simulink model "Car"  (R2016b)
settings: Solver=VariableStepAuto  StartTime=0.0  StopTime=10.0  RelTol=1e-3
settings Model: Creator=Takiya  LastModifiedBy=Takiya

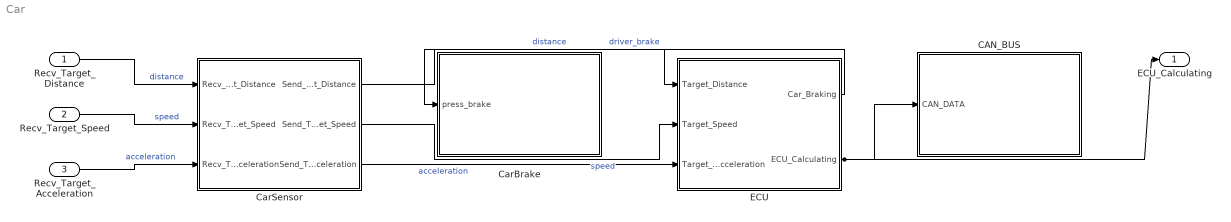
== system Car ==
  Recv_Target_Distance : Inport
      settings: AttributesFormatString=distance
  Recv_Target_Speed : Inport  Port=2
      settings: AttributesFormatString=speed
  Recv_Target_Acceleration : Inport  Port=3
      settings: AttributesFormatString=acceleration
  CAN_BUS : Subsystem
  CarBrake : Subsystem
      settings: AttributesFormatString=Brake
  CarSensor : Subsystem
      settings: AttributesFormatString=Sensor
  ECU : Subsystem
  ECU_Calculating : Outport
  wires:
  CarSensor/3(Send_Target_Acceleration) -> ECU/3(Target_Acceleration)  "acceleration"
  CarSensor/1(Send_Target_Distance) -> ECU/1(Target_Distance)  "distance"
  CarSensor/2(Send_Target_Speed) -> ECU/2(Target_Speed)  "speed"
  ECU/1(Car_Braking) -> CarBrake/1(press_brake)  "driver_brake"
  ECU/2(ECU_Calculating) -> CAN_BUS/1(CAN_DATA), ECU_Calculating/1
  Recv_Target_Distance/1 -> CarSensor/1(Recv_Target_Distance)  "distance"
  Recv_Target_Speed/1 -> CarSensor/2(Recv_Target_Speed)  "speed"
  Recv_Target_Acceleration/1 -> CarSensor/3(Recv_Target_Acceleration)  "acceleration"

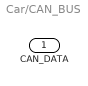
== system Car/CAN_BUS ==
  CAN_DATA : Inport
      settings: AttributesFormatString=ECU_Calculating

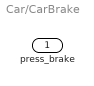
== system Car/CarBrake ==
  press_brake : Inport
      settings: AttributesFormatString=driver_brake

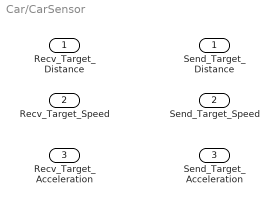
== system Car/CarSensor ==
  Recv_Target_Distance : Inport
      settings: AttributesFormatString=distance
  Recv_Target_Speed : Inport  Port=2
      settings: AttributesFormatString=speed
  Recv_Target_Acceleration : Inport  Port=3
      settings: AttributesFormatString=acceleration
  Send_Target_Distance : Outport
      settings: AttributesFormatString=distance
  Send_Target_Speed : Outport  Port=2
      settings: AttributesFormatString=speed
  Send_Target_Acceleration : Outport  Port=3
      settings: AttributesFormatString=acceleration

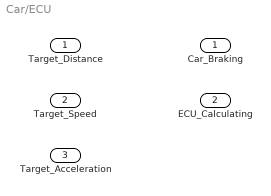
== system Car/ECU ==
  Target_Distance : Inport
      settings: AttributesFormatString=distance
  Target_Speed : Inport  Port=2
      settings: AttributesFormatString=speed
  Target_Acceleration : Inport  Port=3
      settings: AttributesFormatString=acceleration
  Car_Braking : Outport
      settings: AttributesFormatString=driver_brake
  ECU_Calculating : Outport  Port=2
